simulink model "utils"  (Simulink 5.1)
settings: Solver=ode45  StartTime=0.0  StopTime=10.0  RelTol=1e-3
values from neighbouring files (symbols this model uses):
  etaP = 0.75    [Init.m]
  Rb = 0.25/2    (= 0.125)    [Init.m]
  rho = 1.26    [Init.m]
undefined symbols (not defined in the file or in its folder): alpha, Caalpha, eta, lb
settings Model: LastModifiedBy=User  BooleanDataType=on  ProdHWDeviceType=Microprocessor

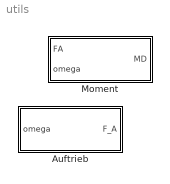
== system utils ==
  Auftrieb : Subsystem
  Moment : Subsystem

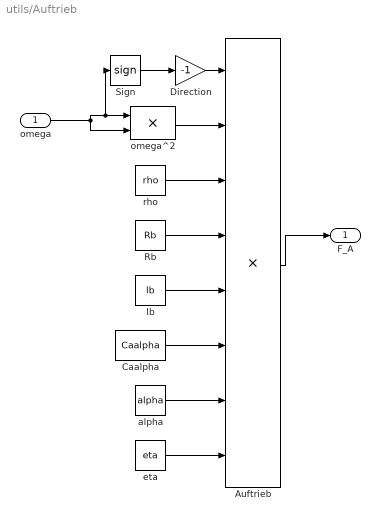
== system utils/Auftrieb ==
  omega : Inport
  Auftrieb : Product  Inputs=8  SaturateOnIntegerOverflow=on
  Caalpha : Constant  Value=Caalpha
  Direction : Gain  Gain=-1  SaturateOnIntegerOverflow=on
  Rb : Constant  Value=Rb
  Sign : Signum
  alpha : Constant  Value=alpha
  eta : Constant  Value=eta
  lb : Constant  Value=lb
  omega^2 : Product  SaturateOnIntegerOverflow=on
  rho : Constant  Value=rho
  F_A : Outport
  wires:
  omega/1 -> omega^2/2, omega^2/1, Sign/1
  omega^2/1 -> Auftrieb/2
  rho/1 -> Auftrieb/3
  Rb/1 -> Auftrieb/4
  lb/1 -> Auftrieb/5
  Caalpha/1 -> Auftrieb/6
  alpha/1 -> Auftrieb/7
  Sign/1 -> Direction/1
  Direction/1 -> Auftrieb/1
  Auftrieb/1 -> F_A/1
  eta/1 -> Auftrieb/8

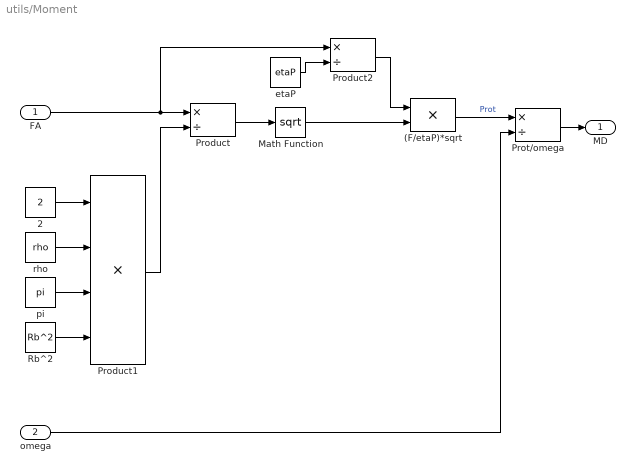
== system utils/Moment ==
  FA : Inport
  omega : Inport  Port=2
  (F/etaP)*sqrt : Product  SaturateOnIntegerOverflow=on
  2 : Constant  Value=2
  Math Function : Math  Operator=sqrt
  Product : Product  Inputs=*/  SaturateOnIntegerOverflow=on
  Product1 : Product  Inputs=4  SaturateOnIntegerOverflow=on
  Product2 : Product  Inputs=*/  SaturateOnIntegerOverflow=on
  Prot/omega : Product  Inputs=*/  SaturateOnIntegerOverflow=on
  Rb^2 : Constant  Value=Rb^2
  etaP : Constant  Value=etaP
  pi : Constant  Value=pi
  rho : Constant  Value=rho
  MD : Outport
  wires:
  FA/1 -> Product/1, Product2/1
  2/1 -> Product1/1
  rho/1 -> Product1/2
  Rb^2/1 -> Product1/4
  pi/1 -> Product1/3
  Product1/1 -> Product/2
  Product/1 -> Math Function/1
  etaP/1 -> Product2/2
  Product2/1 -> (F/etaP)*sqrt/1
  Math Function/1 -> (F/etaP)*sqrt/2
  (F/etaP)*sqrt/1 -> Prot/omega/1  "Prot"
  omega/1 -> Prot/omega/2
  Prot/omega/1 -> MD/1
